simulink model "repo2_6"  (R2019a)
settings: Solver=VariableStepAuto  StartTime=0.0  StopTime=10.0  RelTol=1e-3
settings Model: Creator=toshi  LastModifiedBy=toshi

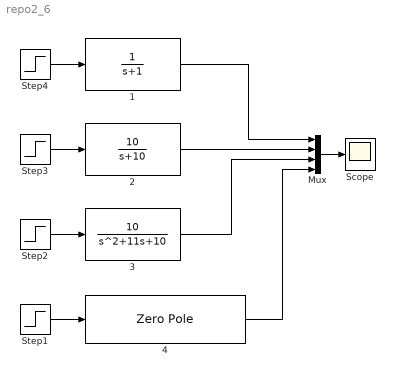
== system repo2_6 ==
  1 : TransferFcn  Denominator=[1 1]
  2 : TransferFcn  Numerator=[10]  Denominator=[1 10]
  3 : TransferFcn  Numerator=[10]  Denominator=[1 11 10]
  4 : ZeroPole  Zeros=[-0.95]  Poles=[-1 -10]  Gain=[10/0.95]
  Mux : Mux
  Scope : Scope
  Step{1..4} (4 alike) : Step  SampleTime=0
  wires:
  Step4/1 -> 1/1
  Step1/1 -> 4/1
  Step2/1 -> 3/1
  Step3/1 -> 2/1
  1/1 -> Mux/1
  2/1 -> Mux/2
  3/1 -> Mux/3
  4/1 -> Mux/4
  Mux/1 -> Scope/1
